simulink model "aquabot_main"  (R2023b)
settings: Solver=FixedStepAuto  StartTime=0.0  StopTime=Inf  RelTol=1e-3
model workspace (MAT data in the model file):
  SL_Bus_ROSEnable64bitIntegers = 1
  SL_ROS_VariableLengthArrays_MaxSizes.CommonInfo.ArrayTruncateAction = 'EmitWarning'
  SL_ROS_VariableLengthArrays_MaxSizes.MsgTypeMap = containers.Map
  SL_ROS_VariableLengthArrays_MaxSizes.MsgTypeMap.serialization.keys = {'nav_msgs/OccupancyGrid', 'sensor_msgs/Image', 'sensor_msgs/LaserScan', 'sensor_msgs/PointCloud2'}
  SL_ROS_VariableLengthArrays_MaxSizes.MsgTypeMap.serialization.values{1}.PropertyName = 'data'
  SL_ROS_VariableLengthArrays_MaxSizes.MsgTypeMap.serialization.values{1}.DataType = 'int8'
  SL_ROS_VariableLengthArrays_MaxSizes.MsgTypeMap.serialization.values{1}.MaxLength = 422500
  SL_ROS_VariableLengthArrays_MaxSizes.MsgTypeMap.serialization.values{2}(1).PropertyName = 'data'
  SL_ROS_VariableLengthArrays_MaxSizes.MsgTypeMap.serialization.values{2}(1).DataType = 'uint8'
  SL_ROS_VariableLengthArrays_MaxSizes.MsgTypeMap.serialization.values{2}(1).MaxLength = 1244160
  SL_ROS_VariableLengthArrays_MaxSizes.MsgTypeMap.serialization.values{2}(2).PropertyName = 'encoding'
  SL_ROS_VariableLengthArrays_MaxSizes.MsgTypeMap.serialization.values{2}(2).DataType = 'uint8'
  SL_ROS_VariableLengthArrays_MaxSizes.MsgTypeMap.serialization.values{2}(2).MaxLength = 1244160
  SL_ROS_VariableLengthArrays_MaxSizes.MsgTypeMap.serialization.values{3}(1).PropertyName = 'intensities'
  SL_ROS_VariableLengthArrays_MaxSizes.MsgTypeMap.serialization.values{3}(1).DataType = 'single'
  SL_ROS_VariableLengthArrays_MaxSizes.MsgTypeMap.serialization.values{3}(1).MaxLength = 1875
  SL_ROS_VariableLengthArrays_MaxSizes.MsgTypeMap.serialization.values{3}(2).PropertyName = 'ranges'
  SL_ROS_VariableLengthArrays_MaxSizes.MsgTypeMap.serialization.values{3}(2).DataType = 'single'
  SL_ROS_VariableLengthArrays_MaxSizes.MsgTypeMap.serialization.values{3}(2).MaxLength = 1875
  SL_ROS_VariableLengthArrays_MaxSizes.MsgTypeMap.serialization.values{4}(1).PropertyName = 'data'
  SL_ROS_VariableLengthArrays_MaxSizes.MsgTypeMap.serialization.values{4}(1).DataType = 'uint8'
  SL_ROS_VariableLengthArrays_MaxSizes.MsgTypeMap.serialization.values{4}(1).MaxLength = 960000
  SL_ROS_VariableLengthArrays_MaxSizes.MsgTypeMap.serialization.values{4}(2).PropertyName = 'fields'
  SL_ROS_VariableLengthArrays_MaxSizes.MsgTypeMap.serialization.values{4}(2).DataType = 'sensor_msgs/PointField'
  SL_ROS_VariableLengthArrays_MaxSizes.MsgTypeMap.serialization.values{4}(2).MaxLength = 16
  SL_ROS_VariableLengthArrays_MaxSizes.MsgTypeMap.serialization.uniformity = 0
  SL_ROS_VariableLengthArrays_MaxSizes.MsgTypeMap.serialization.keyType = 'char'
  SL_ROS_VariableLengthArrays_MaxSizes.MsgTypeMap.serialization.valueType = 'any'
undefined symbols (not defined in the file or in its folder): pose
libraries: ros2lib x16, simulink x1
settings Model: Creator=nicolas  LastModifiedBy=nicolas
settings OptimizationCC: EnhancedBackFolding=on  PassReuseOutputArgsAs=Individual arguments  ZeroExternalMemoryAtStartup=off  ZeroInternalMemoryAtStartup=off  MaxStackSize=64  OptimizeBlockOrder=speed  DifferentSizesBufferReuse=on  OptimizationCustomize=off  EfficientTunableParamExpr=on
settings DebuggingCC: ParameterTunabilityLossMsg=error
settings HardwareCC: ProdBitPerLong=64  ProdLongLongMode=on  ProdHWDeviceType=Intel->x86-64 (Linux 64)  UseEmbeddedCoderFeatures=off
settings SFSimCC: SimHardwareAcceleration=native  SimTargetLang=C++  SimGPUStackLimitPerThread=2048
settings RTWCC: Description=Embedded Coder  SystemTargetFile=ert.tlc  HardwareBoard=Robot Operating System 2 (ROS 2)  TLCOptions="-aInlineSetEventsForThisBaseRateFcn=TLC_FALSE -aSuppressMultiTaskScheduler=TLC_FALSE  -aRateBasedStepFcn=0"  TemplateMakefile=ert_default_tmf  Toolchain=Colcon Tools  BuildConfiguration=Faster Runs  TargetLang=C++
settings CodeAppCC: ForceParamTrailComments=on  IgnoreCustomStorageClasses=off  OperatorAnnotations=on  SimulinkDataObjDesc=on  SFDataObjDesc=on  InsertBlockDesc=on
settings ERTTargetCC: CodeInterfacePackaging=C++ class  SupportNonInlinedSFcns=on  RootIOFormat=Structure reference

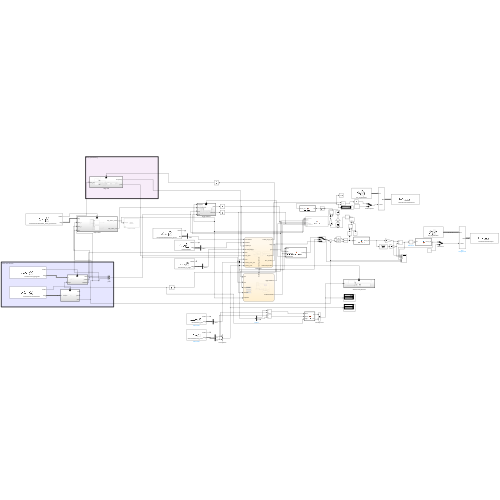
[thumbnail: Simulink's stored preview of the top-level diagram]
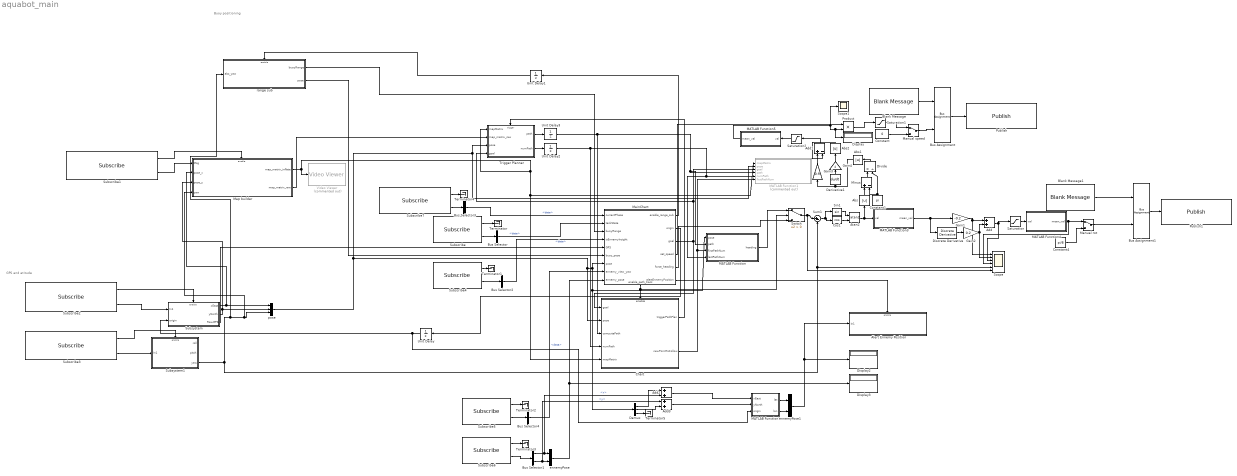
== system aquabot_main ==
  note: Buoy positioning
  note: GPS and atitude
  Abs : Abs  SaturateOnIntegerOverflow=off
  Abs1 : Abs  SaturateOnIntegerOverflow=off
  Abs2 : Abs  SaturateOnIntegerOverflow=off
  Add : Sum
  Add1 : Sum  Inputs=+-
  Add2 : Sum
  Add3 : Sum
  Alert Ennemy Position : Subsystem
  Atan2 : Trigonometry  Operator=atan2
  Blank Message : ros2lib/Blank Message  messageClass=Message  entityType=std_msgs/Float64  messageType=std_msgs/Float64  SampleTime=inf
  Blank Message1 : ros2lib/Blank Message  messageClass=Message  entityType=std_msgs/Float64  messageType=std_msgs/Float64  SampleTime=inf
  Bus Assignment : BusAssignment  AssignedSignals=data
  Bus Assignment1 : BusAssignment  AssignedSignals=data
  Bus Selector{,2..4} (4 alike) : BusSelector  OutputSignals=data
  Bus Selector1 : BusSelector  OutputSignals=pose.position.x,pose.position.y
  Chart : Stateflow chart  TreatAsAtomicUnit=on
      settings: PortSchema="{\"entries\":[{\"content\":{\"sides\":[{\"content\":{\"connectorIds\":[\"In2\",\"In3\",\"In4\",\"In5\",\"In6\"]},\"type\":\"ConnectorPlacement.EquallySpacedRectSide\",\"uuid\":\"f9d23542-f88c-4b93-885e-55d9e7a867a5\"},{\"content\":{\"connectorIds\":[\"Out1\",\"Out2\"],\"side\":\"RIGHT\"},\"type\":\"ConnectorPlacement.EquallySpacedRectSide\",\"uuid\":\"ec7f353a-44e5-4b1c-b599-993baee30662\"},{\"content\":{\"connectorIds\":[\"In1\"],\"side\":\"TOP\"},\"type\":\"ConnectorPlacement.EquallySpacedRectSide\",\"uuid\":\"e2b72665-f6a6-46cc-93cf-7087a3433fd3\"}]},\"type\":\"ConnectorPlacement.EquallySpacedConnector\",\"uuid\":\"eb72d472-900e-4b4b-88a5-7b3bc966b645\"}],\"packageUris\":[\"http://schema.mathworks.com/mf0/Connector/R2020b\"],\"version\":\"1.0\"}"
  Constant : Constant  Value=0
  Constant1 : Constant  Value=pi
  Constant4 : Constant  Value=pi/8
  Cos1 : Trigonometry  Operator=cos
  Demux : Demux  Outputs=3
  Derivative1 : Derivative
  Discrete Derivative : simulink/Discrete/Discrete Derivative  gainval=1.0  ICPrevScaledInput=0.0  OutMin=[]  OutMax=[]  OutDataType=fixdt(1, 16)  OutScaling=2^-10  DoSatur=off
  Display : Display
  Display2 : Display
  Display3 : Display
  Divide : Product  Inputs=*/  RndMeth=Zero  SaturateOnIntegerOverflow=on
  Gain1 : Gain  Gain=-0.2
  Gain2 : Gain  Gain=0.2
  Gain3 : Gain  Gain=0.9
  Gain4 : Gain  Gain=4
  MATLAB Function : MATLAB Function  TreatAsAtomicUnit=on
  MATLAB Function1 : MATLAB Function  Commented=on  TreatAsAtomicUnit=on
  MATLAB Function2 : MATLAB Function  TreatAsAtomicUnit=on
  MATLAB Function3 : MATLAB Function  TreatAsAtomicUnit=on
  MATLAB Function4 : MATLAB Function  TreatAsAtomicUnit=on
  MATLAB Function5 : MATLAB Function  TreatAsAtomicUnit=on
  MainChart : Stateflow chart  TreatAsAtomicUnit=on
      settings: PortSchema="{\"entries\":[{\"content\":{\"sides\":[{\"content\":{\"connectorIds\":[\"In9\",\"In1\",\"In2\",\"In3\",\"In4\",\"In5\",\"In6\",\"In7\",\"In8\"]},\"type\":\"ConnectorPlacement.EquallySpacedRectSide\",\"uuid\":\"baf46242-21ef-496b-8046-9b9a77bd2dcf\"},{\"content\":{\"connectorIds\":[\"Out1\",\"Out2\",\"Out3\",\"Out4\",\"Out6\",\"Out7\"],\"side\":\"RIGHT\"},\"type\":\"ConnectorPlacement.EquallySpacedRectSide\",\"uuid\":\"0a7db7ae-9b8c-430e-84d2-7611729502e6\"},{\"content\":{\"side\":\"TOP\"},\"type\":\"ConnectorPlacement.EquallySpacedRectSide\",\"uuid\":\"959f44e0-4ee3-46d3-b72a-0b37b61c16dd\"},{\"content\":{\"connectorIds\":[\"Out5\"],\"side\":\"BOTTOM\"},\"type\":\"ConnectorPlacement.EquallySpacedRectSide\",\"uuid\":\"d94f5cc5-2498-45e0-a229-1de127971452\"}]},\"type\":\"ConnectorPlacement.EquallySpacedConnector\",\"uuid\":\"f5cd4cf7-e63f-491e-bc4b-a2135ba07ed7\"}],\"packageUris\":[\"http://schema.mathworks.com/mf0/Connector/R2020b\"],\"version\":\"1.0\"}"
  Manual rot : ManualSwitch
  Manual speed : ManualSwitch
  Map builder : Subsystem
  Minus : Sum  Inputs=+-
  Product : Product
  Publish : ros2lib/Publish  topicSource=Select from ROS network  topic=/wamv/thrusters/main/thrust  messageType=std_msgs/Float64  QOSHistory=Keep last  QOSDepth=1  QOSReliability=Reliable  QOSDurability=Volatile
  Publish1 : ros2lib/Publish  topicSource=Select from ROS network  topic=/wamv/thrusters/main/pos  messageType=std_msgs/Float64  QOSHistory=Keep last  QOSDepth=1  QOSReliability=Reliable  QOSDurability=Volatile
  Saturation : Saturate  UpperLimit=pi/4  LowerLimit=-pi/4
  Saturation1 : Saturate  UpperLimit=12000  LowerLimit=-12000
  Saturation2 : Saturate  UpperLimit=1  LowerLimit=0.1
  Scope : Scope  NumInputPorts=6
  Scope1 : Scope
  Sin1 : Trigonometry
  Subscribe : ros2lib/Subscribe  topicSource=Select from ROS network  topic=/siera/task/state  messageType=std_msgs/Int64  sampleTime=-1  QOSHistory=Keep last  QOSDepth=1  QOSReliability=Reliable  QOSDurability=Volatile
  Subscribe1 : ros2lib/Subscribe  topicSource=Select from ROS network  topic=/wamv/sensors/lidars/lidar_wamv_sensor/scan  messageType=sensor_msgs/LaserScan  sampleTime=-1  QOSHistory=Keep last  QOSDepth=1  QOSReliability=Reliable  QOSDurability=Volatile
  Subscribe2 : ros2lib/Subscribe  topicSource=Select from ROS network  topic=/wamv/sensors/gps/gps/fix  messageType=sensor_msgs/NavSatFix  sampleTime=-1  QOSHistory=Keep last  QOSDepth=1  QOSReliability=Reliable  QOSDurability=Volatile
  Subscribe3 : ros2lib/Subscribe  topicSource=Select from ROS network  topic=/wamv/sensors/imu/imu/data  messageType=sensor_msgs/Imu  sampleTime=-1  QOSHistory=Keep last  QOSDepth=1  QOSReliability=Reliable  QOSDurability=Volatile
  Subscribe4 : ros2lib/Subscribe  topicSource=Select from ROS network  topic=/siera/view/is_in_sight  messageType=std_msgs/Bool  sampleTime=-1  QOSHistory=Keep last  QOSDepth=1  QOSReliability=Reliable  QOSDurability=Volatile
  Subscribe5 : ros2lib/Subscribe  topicSource=Select from ROS network  topic=/siera/view/rel_yaw  messageType=std_msgs/Float64  sampleTime=-1  QOSHistory=Keep last  QOSDepth=1  QOSReliability=Reliable  QOSDurability=Volatile
  Subscribe6 : ros2lib/Subscribe  topicSource=Select from ROS network  topic=/siera/view/ennemy_pose  messageType=geometry_msgs/PoseStamped  sampleTime=-1  QOSHistory=Keep last  QOSDepth=1  QOSReliability=Reliable  QOSDurability=Volatile
  Subscribe7 : ros2lib/Subscribe  topicSource=Select from ROS network  topic=/vrx/patrolandfollow/current_phase  messageType=std_msgs/UInt32  sampleTime=-1  QOSHistory=Keep last  QOSDepth=1  QOSReliability=Reliable  QOSDurability=Volatile
  Subsystem : Subsystem
  Subsystem1 : Subsystem
  Sum1 : Sum  Inputs=|+-
  Switch : Switch  Criteria=u2 > Threshold  SaturateOnIntegerOverflow=off  InputSameDT=off
  Terminator{,1..5} (6 alike) : Terminator
  Trigger Planner : Subsystem
  Unit Delay : UnitDelay  InitialCondition=[0 0]  SampleTime=-1  HasFrameUpgradeWarning=on
  Unit Delay1 : UnitDelay  SampleTime=-1  HasFrameUpgradeWarning=on
  Unit Delay2 : UnitDelay  SampleTime=-1  HasFrameUpgradeWarning=on
  Unit Delay3 : UnitDelay  InitialCondition=zeros(100,3)  SampleTime=-1  HasFrameUpgradeWarning=on
  Video Viewer : VideoViewer  Commented=on  FigPos=[317 969 1054 739]
  ennemyPose : Concatenate
  ennemyPose1 : Concatenate
  pose : Concatenate  NumInputs=3
  range sub : Subsystem
  wires:
  Subscribe1/2 -> Map builder/1(Msg)
  Subscribe1/1 -> Map builder/Enable
  Subscribe3/2 -> Subsystem1/1(In1)
  Subscribe3/1 -> Subsystem1/Enable
  Map builder/1(map_matrix_inflate) -> Video Viewer/1, Trigger Planner/1(mapMatrix), Chart/6(mapMatrix), MATLAB Function1/1(mapMatrix)
  Subscribe4/2 -> Bus Selector2/1
  Bus Selector/1 -> MainChart/1(taskState)  "<data>"
  MainChart/1(enable_range_sub) -> Unit Delay1/1
  Blank Message/1 -> Bus Assignment/1
  Bus Assignment/1 -> Publish/1
  Subscribe2/2 -> Subsystem/1(In1)
  MainChart/2(origin) -> Unit Delay/1
  Subsystem/3(RawGPS) -> MainChart/4(GPS)
  Subscribe2/1 -> Subsystem/Enable
  Unit Delay/1 -> MATLAB Function2/3(origin), Subsystem/2(origin)
  Subsystem/1(xEast) -> Map builder/2(pose_x), pose/1
  Subsystem/2(yNorth) -> pose/2, Map builder/3(pose_y)
  pose/1 -> MATLAB Function1/2(pose), Trigger Planner/3(pose), Chart/3(pose), Demux/1, MATLAB Function/1(pose), MainChart/6(pose)
  Unit Delay1/1 -> range sub/Enable
  range sub/2(pose) -> MainChart/5(buoy_pose)
  Trigger Planner/2(numPath) -> Unit Delay2/1
  Chart/1(triggerPathPlan) -> Trigger Planner/Trigger
  Trigger Planner/1(path) -> Unit Delay3/1
  Unit Delay2/1 -> Chart/5(numPath), MATLAB Function1/5(numPath), MATLAB Function/4(lastPathNum)
  Unit Delay3/1 -> Chart/4(computePath), MATLAB Function/2(path), MATLAB Function1/4(path)
  Chart/2(newPointToFollow) -> MATLAB Function/3(firstPathNum), MATLAB Function1/6(firstPathNum)
  Blank Message1/1 -> Bus Assignment1/1
  Bus Assignment1/1 -> Publish1/1
  MATLAB Function/1(heading) -> Switch/1
  MATLAB Function3/1(mean_val) -> Gain1/1, Discrete Derivative/1
  Cos1/1 -> Atan2/2
  Sin1/1 -> Atan2/1
  Atan2/1 -> MATLAB Function3/1(val), Abs/1
  Sum1/1 -> Sin1/1, Cos1/1
  Gain2/1 -> Scope/2, Add/2
  Gain1/1 -> Add/1, Scope/1
  Saturation/1 -> MATLAB Function4/1(val)
  Add/1 -> Saturation/1, Scope/3
  MainChart/4(set_speed) -> Product/1
  Manual speed/1 -> Bus Assignment/2
  Constant/1 -> Manual speed/2
  Constant4/1 -> Manual rot/2
  Manual rot/1 -> Bus Assignment1/2
  Subsystem1/3(yaw) -> pose/3, Map builder/4(yaw), range sub/1(abs_yaw), Sum1/2, Scope/5
  range sub/1(buoyRange) -> MainChart/2(buoyRange)
  MainChart/3(goal) -> Chart/2(goal), MATLAB Function1/3(goal), Trigger Planner/4(goal)
  MainChart/5(enable_path_track) -> Switch/2, Chart/1(enable)
  Abs/1 -> Minus/1
  Constant1/1 -> Minus/2, Divide/2
  Minus/1 -> Divide/1
  Divide/1 -> Abs1/1
  Saturation1/1 -> Manual speed/1
  Product/1 -> Saturation1/1
  MATLAB Function5/1(mean_val) -> Display/1, Product/2, Scope1/1
  Derivative1/1 -> Gain4/1
  Add1/1 -> Saturation2/1
  Gain3/1 -> Add1/1
  Abs1/1 -> Gain3/1, Derivative1/1
  Gain4/1 -> Abs2/1
  Abs2/1 -> Add1/2
  Subscribe/2 -> Bus Selector/1
  Subscribe/1 -> Terminator/1
  Switch/1 -> Scope/6, Sum1/1
  MainChart/6(force_heading) -> Switch/3
  Subscribe4/1 -> Terminator1/1
  Subscribe5/1 -> Terminator2/1
  Subscribe6/2 -> Bus Selector1/1
  Subscribe6/1 -> Terminator3/1
  Bus Selector1/2 -> Add3/1, ennemyPose/2  "<y>"
  Bus Selector1/1 -> Add2/2, ennemyPose/1  "<x>"
  Subscribe5/2 -> Bus Selector4/1
  ennemyPose/1 -> Display3/1, MainChart/8(ennemy_pose)
  Subscribe7/1 -> Terminator4/1
  Subscribe7/2 -> Bus Selector3/1
  MainChart/7(alertEnnemyPosition) -> Alert Ennemy Position/Enable
  Bus Selector2/1 -> MainChart/3(isEnnemyInsight)  "<data>"
  Bus Selector3/1 -> MainChart/9(currentPhase)  "<data>"
  Bus Selector4/1 -> MainChart/7(ennemy_view_yaw)  "<data>"
  MATLAB Function2/1(lat) -> ennemyPose1/1
  MATLAB Function2/2(lon) -> ennemyPose1/2
  ennemyPose1/1 -> Alert Ennemy Position/1(In1), Display2/1
  MATLAB Function4/1(mean_val) -> Scope/4, Manual rot/1
  Discrete Derivative/1 -> Gain2/1
  Saturation2/1 -> MATLAB Function5/1(val)
  Add2/1 -> MATLAB Function2/1(xEast)
  Add3/1 -> MATLAB Function2/2(yNorth)
  Demux/1 -> Add2/1
  Demux/2 -> Add3/2
  Demux/3 -> Terminator5/1
  Map builder/2(map_matrix_raw) -> Trigger Planner/2(map_matrix_raw)

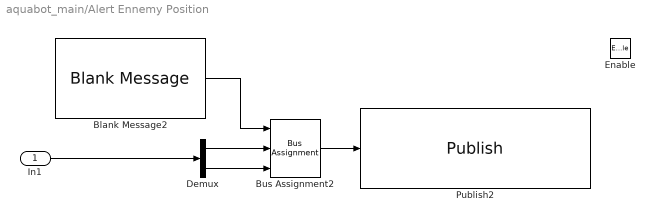
== system aquabot_main/Alert Ennemy Position ==
  In1 : Inport
  Enable : EnablePort
  Blank Message2 : ros2lib/Blank Message  messageClass=Message  entityType=geometry_msgs/PoseStamped  messageType=geometry_msgs/PoseStamped  SampleTime=inf
  Bus Assignment2 : BusAssignment  AssignedSignals=pose.position.x,pose.position.y
  Demux : Demux  Outputs=2
  Publish2 : ros2lib/Publish  topicSource=Select from ROS network  topic=/vrx/patrolandfollow/alert_position  messageType=geometry_msgs/PoseStamped  QOSHistory=Keep last  QOSDepth=1  QOSReliability=Reliable  QOSDurability=Volatile
  wires:
  In1/1 -> Demux/1
  Demux/1 -> Bus Assignment2/2
  Bus Assignment2/1 -> Publish2/1
  Blank Message2/1 -> Bus Assignment2/1
  Demux/2 -> Bus Assignment2/3

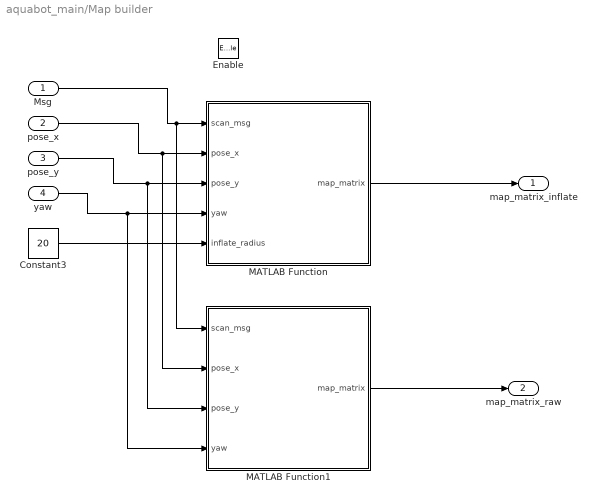
== system aquabot_main/Map builder ==
  Msg : Inport
  pose_x : Inport  Port=2
  pose_y : Inport  Port=3
  yaw : Inport  Port=4
  Enable : EnablePort
  Constant3 : Constant  Value=20
  MATLAB Function : MATLAB Function  TreatAsAtomicUnit=on
  MATLAB Function1 : MATLAB Function  TreatAsAtomicUnit=on
  map_matrix_inflate : Outport
  map_matrix_raw : Outport  Port=2
  wires:
  Msg/1 -> MATLAB Function1/1(scan_msg), MATLAB Function/1(scan_msg)
  MATLAB Function/1(map_matrix) -> map_matrix_inflate/1
  pose_x/1 -> MATLAB Function1/2(pose_x), MATLAB Function/2(pose_x)
  pose_y/1 -> MATLAB Function1/3(pose_y), MATLAB Function/3(pose_y)
  yaw/1 -> MATLAB Function1/4(yaw), MATLAB Function/4(yaw)
  Constant3/1 -> MATLAB Function/5(inflate_radius)
  MATLAB Function1/1(map_matrix) -> map_matrix_raw/1

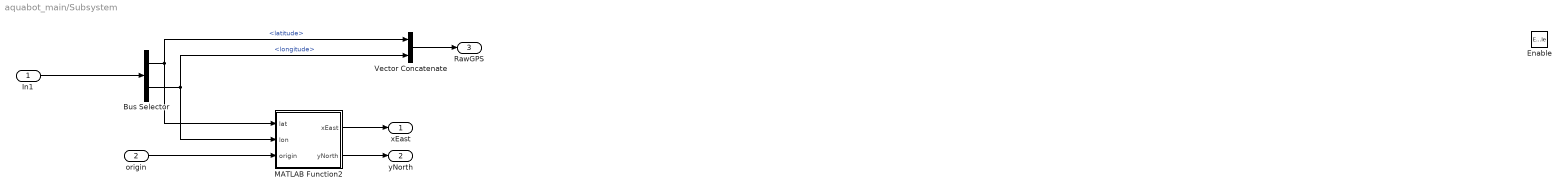
== system aquabot_main/Subsystem ==
  In1 : Inport
  origin : Inport  Port=2
  Enable : EnablePort
  Bus Selector : BusSelector  OutputSignals=latitude,longitude
  MATLAB Function2 : MATLAB Function  TreatAsAtomicUnit=on
  Vector Concatenate : Concatenate
  xEast : Outport
  yNorth : Outport  Port=2
  RawGPS : Outport  Port=3
  wires:
  In1/1 -> Bus Selector/1
  Bus Selector/1 -> MATLAB Function2/1(lat), Vector Concatenate/1  "<latitude>"
  Vector Concatenate/1 -> RawGPS/1
  Bus Selector/2 -> MATLAB Function2/2(lon), Vector Concatenate/2  "<longitude>"
  origin/1 -> MATLAB Function2/3(origin)
  MATLAB Function2/1(xEast) -> xEast/1
  MATLAB Function2/2(yNorth) -> yNorth/1

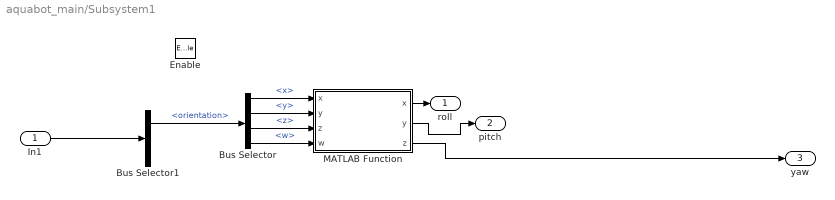
== system aquabot_main/Subsystem1 ==
  In1 : Inport
  Enable : EnablePort
  Bus Selector : BusSelector  OutputSignals=x,y,z,w
  Bus Selector1 : BusSelector  OutputSignals=orientation,angular_velocity
  MATLAB Function : MATLAB Function  TreatAsAtomicUnit=on
  roll : Outport
  pitch : Outport  Port=2
  yaw : Outport  Port=3
  wires:
  Bus Selector1/1 -> Bus Selector/1  "<orientation>"
  Bus Selector/2 -> MATLAB Function/2("y ")  "<y>"
  Bus Selector/4 -> MATLAB Function/4(w)  "<w>"
  Bus Selector/3 -> MATLAB Function/3("z ")  "<z>"
  MATLAB Function/2(y) -> pitch/1
  Bus Selector/1 -> MATLAB Function/1("x ")  "<x>"
  In1/1 -> Bus Selector1/1
  MATLAB Function/3(z) -> yaw/1
  MATLAB Function/1(x) -> roll/1

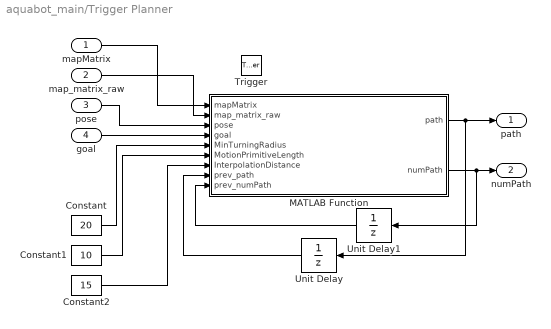
== system aquabot_main/Trigger Planner ==
  mapMatrix : Inport
  map_matrix_raw : Inport  Port=2
  pose : Inport  Port=3
  goal : Inport  Port=4
  Trigger : TriggerPort  VariantControl=(inherit)  PortDimensions=1
  Constant : Constant  Value=20
  Constant1 : Constant  Value=10
  Constant2 : Constant  Value=15
  MATLAB Function : MATLAB Function  TreatAsAtomicUnit=on
  Unit Delay : UnitDelay  InitialCondition=zeros(100,3)  SampleTime=-1  HasFrameUpgradeWarning=on
  Unit Delay1 : UnitDelay  InitialCondition=1  SampleTime=-1  HasFrameUpgradeWarning=on
  path : Outport
  numPath : Outport  Port=2
  wires:
  goal/1 -> MATLAB Function/4(goal)
  pose/1 -> MATLAB Function/3(pose)
  MATLAB Function/2(numPath) -> Unit Delay1/1, numPath/1
  mapMatrix/1 -> MATLAB Function/1(mapMatrix)
  MATLAB Function/1(path) -> Unit Delay/1, path/1
  Constant2/1 -> MATLAB Function/7(InterpolationDistance)
  Constant1/1 -> MATLAB Function/6(MotionPrimitiveLength)
  Constant/1 -> MATLAB Function/5(MinTurningRadius)
  Unit Delay/1 -> MATLAB Function/8(prev_path)
  Unit Delay1/1 -> MATLAB Function/9(prev_numPath)
  map_matrix_raw/1 -> MATLAB Function/2(map_matrix_raw)

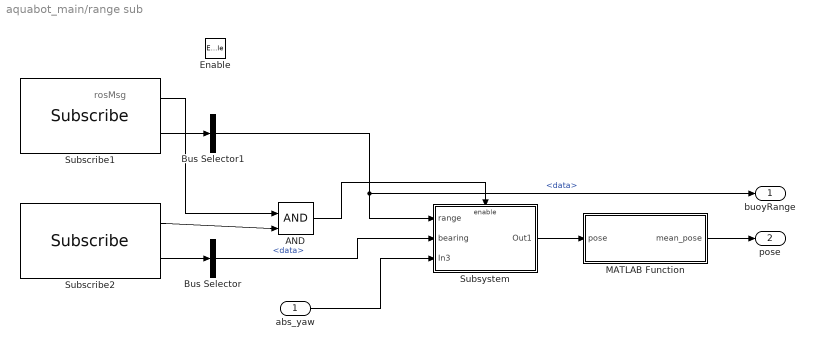
== system aquabot_main/range sub ==
  note: rosMsg
  abs_yaw : Inport
  Enable : EnablePort
  AND : Logic  IconShape=distinctive  AllPortsSameDT=off  OutDataTypeStr=boolean
  Bus Selector : BusSelector  OutputSignals=data
  Bus Selector1 : BusSelector  OutputSignals=data
  MATLAB Function : MATLAB Function  TreatAsAtomicUnit=on
  Subscribe1 : ros2lib/Subscribe  topicSource=Select from ROS network  topic=/siera/pinger/range  messageType=std_msgs/Float64  sampleTime=-1  QOSHistory=Keep last  QOSDepth=1  QOSReliability=Reliable  QOSDurability=Volatile
  Subscribe2 : ros2lib/Subscribe  topicSource=Select from ROS network  topic=/siera/pinger/bearing  messageType=std_msgs/Float64  sampleTime=-1  QOSHistory=Keep last  QOSDepth=1  QOSReliability=Reliable  QOSDurability=Volatile
  Subsystem : Subsystem
  buoyRange : Outport
  pose : Outport  Port=2
  wires:
  Subscribe1/2 -> Bus Selector1/1
  Subscribe2/2 -> Bus Selector/1
  Subscribe2/1 -> AND/2
  Subscribe1/1 -> AND/1
  Bus Selector1/1 -> buoyRange/1, Subsystem/1(range)  "<data>"
  Bus Selector/1 -> Subsystem/2(bearing)  "<data>"
  abs_yaw/1 -> Subsystem/3(In3)
  Subsystem/1(Out1) -> MATLAB Function/1(pose)
  AND/1 -> Subsystem/Enable
  MATLAB Function/1(mean_pose) -> pose/1

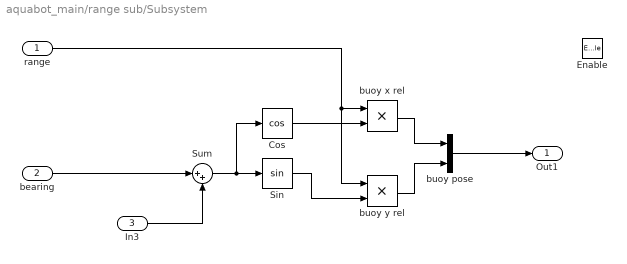
== system aquabot_main/range sub/Subsystem ==
  range : Inport
  bearing : Inport  Port=2
  In3 : Inport  Port=3
  Enable : EnablePort
  Cos : Trigonometry  Operator=cos
  Sin : Trigonometry
  Sum : Sum  Inputs=|++
  buoy pose : Concatenate
  buoy x rel : Product
  buoy y rel : Product
  Out1 : Outport
  wires:
  Cos/1 -> buoy x rel/2
  In3/1 -> Sum/2
  buoy pose/1 -> Out1/1
  Sin/1 -> buoy y rel/2
  buoy x rel/1 -> buoy pose/1
  buoy y rel/1 -> buoy pose/2
  range/1 -> buoy y rel/1, buoy x rel/1
  Sum/1 -> Cos/1, Sin/1
  bearing/1 -> Sum/1

== matlab function aquabot_main/Map builder/MATLAB Function ==
  data: scan_msg input; map_matrix output; pose_x input; pose_y input; yaw input; inflate_radius input
function map_matrix= fcn(scan_msg, pose_x, pose_y, yaw,inflate_radius)
    ranges = scan_msg.ranges;
    ranges(ranges==inf) = NaN;
    angles = transpose(linspace(scan_msg.angle_min, scan_msg.angle_max, length(ranges)));

    map = binaryOccupancyMap(700, 700,1);
    map.GridOriginInLocal = -[diff(map.XWorldLimits) diff(map.YWorldLimits)]/2;
    insertRay(map, [pose_x pose_y yaw], ranges, angles, 130);
    inflate(map,inflate_radius)
    map_matrix = map.occupancyMatrix();
end

== matlab function aquabot_main/Subsystem1/MATLAB Function ==
  data: x output; x input; y output; y input; z input; w input; z output
function [x, y, z]= quatToEuler(x, y, z, w)
    eulZYX = quat2eul([w, x, y, z], "ZYX");
    x = eulZYX(3);
    y = eulZYX(2);
    z = eulZYX(1);
end

== stateflow chart aquabot_main/MainChart ==
  state Init
    entry:
    goal = [0; 0];
    set_speed=0;
    enable_path_track = 0;
    force_heading = pose(3);
    listOfPoints = [[200;200],[200;-200],[0;200],[0;-200],[-200;200],[-200;-200]];
  state SeekBuoy
    entry:
    origin = [GPS(1); GPS(2)];
    force_heading = pose(3);
    enable_range_sub=1;
    set_speed=8000;
    enable_path_track = 1;
    during:
    new_goal = [buoy_pose(1) + pose(1); buoy_pose(2) + pose(2)];
    goal = (new_goal + goal) / 2;
  state FineBuoySeeking
    entry:
    set_speed=2000;
    force_heading = pose(3);
    enable_path_track = 0;
    during:
    force_heading = atan2(goal(2)-pose(2), goal(1)-pose(1));
  state BuoyFound
    entry:
    set_speed=2000;
    force_heading = pose(3);
    enable_path_track = 0;
    during:
    force_heading = atan2(-goal(2)-pose(2), -goal(1)-pose(1));
  state Patroll
    entry:
    set_speed=0;
    enable_range_sub=0;
    state Init
    state FollowGoal
      entry:
      set_speed=10000;
      goal = listOfPoints(:,indexOfNextGoal);
      enable_path_track = 1;
    state GoalAchieve
      entry:
      indexOfNextGoal = mod(indexOfNextGoal, size(listOfPoints,2))+1;
    (default) -> Patroll.Init
    Patroll.Init -> FollowGoal
    GoalAchieve -> FollowGoal
    FollowGoal -> GoalAchieve : [norm(goal - pose(1:2)) <= 10]
  state SeekEnnemy
    entry:
    set_speed=0;
    state SeekInSight
      entry:
      set_speed=5000;
      enable_path_track = 1;
      during:
      force_heading = pose(3) - ennemy_view_yaw;
      goal = pose(1:2) + [80 * cos(pose(3) - ennemy_view_yaw); 80*sin(pose(3)) - ennemy_view_yaw ];
    state SearchLastKnowZone
      set_speed=3000;
      enable_path_track = 1;
    state EnnemyOnLidar
      entry:
      enable_path_track = 1;
      alertEnnemyPosition=1;
      during:
      % force_heading = pose(3) - ennemy_view_yaw;
      goal = pose(1:2) + ennemy_pose;
      distance = norm(goal - pose(1:2));
      set_speed = max(min((distance-30)*30,3000),0);
    (default) -> SeekInSight
    SeekInSight -> SearchLastKnowZone [order 1] : [isEnnemyInsight==0]
    (junction 177) -> SeekInSight [order 1] : [isEnnemyInsight==1]
    SearchLastKnowZone -> SeekInSight [order 2] : [isEnnemyInsight==1]
    SeekInSight -> EnnemyOnLidar [order 2] : [all(ennemy_pose)~=0]
    SearchLastKnowZone -> EnnemyOnLidar [order 1] : [all(ennemy_pose)~=0]
    SearchLastKnowZone -> (junction 177) [order 3] : [norm(goal - pose(1:2)) <= 5]
    EnnemyOnLidar -> SearchLastKnowZone : [all(ennemy_pose)==0]{alertEnnemyPosition=0;}
  state TurnAroundToSeekNearEnnemy
    entry:
    start_yaw = pose(3);
    force_heading = start_yaw;
    during:
    force_heading = force_heading + 0.002;
  (default) -> Init
  Init -> SeekBuoy : [taskState==2 && all(GPS)~=0]
  SeekBuoy -> FineBuoySeeking : [buoyRange<=40||currentPhase>=2]
  FineBuoySeeking -> BuoyFound : [buoyRange<=20||currentPhase>=2]
  Patroll -> SeekEnnemy : [isEnnemyInsight==1]
  TurnAroundToSeekNearEnnemy -> Patroll [order 1] : [force_heading-start_yaw>=2*pi]
  BuoyFound -> TurnAroundToSeekNearEnnemy : [currentPhase>=2]{indexOfNextGoal = 1;}
  (junction 177) -> TurnAroundToSeekNearEnnemy [order 2] : after(50,sec)
  TurnAroundToSeekNearEnnemy -> SeekEnnemy [order 2] : [isEnnemyInsight==1]
  data: taskState input; buoyRange input; isEnnemyInsight input; enable_range_sub output; origin output; GPS input; buoy_pose input; pose input; goal output; new_goal local; set_speed output; enable_path_track output; force_heading output; listOfPoints local; indexOfNextGoal local; ennemy_view_yaw input; ennemy_pose input; alertEnnemyPosition output; currentPhase input; start_yaw local; distance local

== matlab function aquabot_main/MATLAB Function2 ==
  data: lat output; lon output; xEast input; yNorth input; origin input
function [lat,lon] = XY2GPS(xEast,yNorth, origin)
    earth_radius = 6371000.0;
    
    if all(origin == 0)
        lat = 0;
        lon = 0;
    else
        lat = rad2deg(asin(yNorth/earth_radius)) + origin(1);
        lon = rad2deg(asin(xEast/(earth_radius*cos(asin(yNorth/earth_radius))))) + origin(2);
    end
end

== matlab function aquabot_main/MATLAB Function3 ==
  data: val input; mean_val output
function mean_val = movMean(val)
    persistent vals;
    persistent lastValIndex;    
    mov_length = 10;
    
    if isempty(vals)
        vals = zeros(mov_length,1);
        lastValIndex = 1;
    end

    vals = circshift(vals, [-1 0]);
    vals(lastValIndex) = val;

    mean_val = mean(vals(1:lastValIndex,:));
    if lastValIndex < mov_length
        lastValIndex = lastValIndex + 1;
    end
end

== matlab function aquabot_main/Trigger Planner/MATLAB Function ==
  data: mapMatrix input; map_matrix_raw input; path output; numPath output; pose input; goal input; MinTurningRadius input; MotionPrimitiveLength input; InterpolationDistance input; prev_path input; prev_numPath input
function [path, numPath] = planner(mapMatrix, map_matrix_raw, pose, goal, MinTurningRadius, MotionPrimitiveLength, InterpolationDistance, prev_path, prev_numPath)
    persistent prev_goal;
    MaxPathNum = 100;

    if isempty(prev_goal)
        prev_goal = goal;
    end

    map = binaryOccupancyMap(mapMatrix, 1);
    map.GridOriginInLocal = -[diff(map.XWorldLimits) diff(map.YWorldLimits)]/2;
    
    ss = stateSpaceSE2;
    ss.StateBounds = [map.XWorldLimits;map.YWorldLimits;[-pi pi]];
    if isempty(ss)
        path = prev_path;
        numPath = prev_numPath;
        return;
    end
    sv = validatorOccupancyMap(ss,Map=map);

    planner = plannerHybridAStar(sv, MinTurningRadius=MinTurningRadius, MotionPrimitiveLength=MotionPrimitiveLength, InterpolationDistance=InterpolationDistance);
    startPose = pose'; % [meters, meters, radians]
    goal(1) = min(max(goal(1),-320),320);
    goal(2) = min(max(goal(2),-320),320);
    goalOrientation = atan2(goal(2) - pose(2), goal(1) - pose(1));
    goalPose = [goal(1) goal(2) goalOrientation];
    
    if ~isStateValid(sv,startPose)
        map = binaryOccupancyMap(map_matrix_raw, 1);
        map.GridOriginInLocal = -[diff(map.XWorldLimits) diff(map.YWorldLimits)]/2;
        sv = validatorOccupancyMap(ss,Map=map);
        planner = plannerHybridAStar(sv, MinTurningRadius=MinTurningRadius, MotionPrimitiveLength=MotionPrimitiveLength, InterpolationDistance=InterpolationDistance);
    end

    if ~isStateValid(sv,goalPose)
        [~, lastValid] = isMotionValid(sv,startPose,goalPose);
        goalOrientation = atan2(lastValid(2) - pose(2), lastValid(1) - pose(1));            
        goalPose = [lastValid(1) lastValid(2) goalOrientation];
    end

    if norm(startPose - goalPose) <= 10
        path = zeros(MaxPathNum,3);
        path(1,:) = startPose;
        goalOrientation = atan2(goal(2) - pose(2), goal(1) - pose(1));
        goalPose = [goal(1) goal(2) goalOrientation];
        path(2,:) = goalPose;
        numPath=2;
    else
        refpath = plan(planner,startPose,goalPose);
        path = zeros(MaxPathNum,3);
        path(1:refpath.NumStates,:) = refpath.States;
        numPath=refpath.NumStates;
    end
end

== matlab function aquabot_main/MATLAB Function1 ==
  data: mapMatrix input; pose input; goal input; path input; numPath input; firstPathNum input
function viewDebug(mapMatrix, pose, goal, path, numPath, firstPathNum)
    [r,c] = ind2sub(size(mapMatrix), find(mapMatrix));
    r = 325 - r;
    c = c - 325;
    
    hold off
    scatter(c,r,'filled','square','MarkerFaceColor','k')
    hold on
    plot(pose(1), pose(2), "-o", "MarkerEdgeColor", "g")
    plot(goal(1), goal(2), "-o", "MarkerEdgeColor", "r")
    range = 25;
    quiver(pose(1), pose(2), range*cos(pose(3)), range*sin(pose(3)))

    if numPath > 0
        scatter(path(firstPathNum+1:numPath-1,1),path(firstPathNum+1:numPath-1,2),'o','MarkerFaceColor','b')
        scatter(path(firstPathNum,1),path(firstPathNum,2),'o','MarkerFaceColor','g')
        scatter(path(numPath,1),path(numPath,2),'o','MarkerFaceColor','r')
        range = 5;
        quiver(path(firstPathNum:numPath,1), path(firstPathNum:numPath,2), range*cos(path(firstPathNum:numPath,3)), range*sin(path(firstPathNum:numPath,3)))
    end

    xlim([-325 325])
    ylim([-325 325])
end

== matlab function aquabot_main/Subsystem/MATLAB Function2 ==
  data: xEast output; yNorth output; lat input; lon input; origin input
function [xEast,yNorth] = GPS2XY(lat,lon, origin)
    earth_radius = 6371000.0;
    
    if all(origin == 0)
        xEast = 0;
        yNorth = 0;
    else
        xEast = earth_radius * cos(deg2rad(lat - origin(1))) * sin(deg2rad(lon - origin(2)));
        yNorth = earth_radius * sin(deg2rad(lat - origin(1)));
    end
end

== matlab function aquabot_main/MATLAB Function ==
  data: pose input; path input; heading output; firstPathNum input; lastPathNum input
function heading = convertPathPlanToHeading(pose, path, firstPathNum, lastPathNum)
    persistent prev_heading;
    if isempty(prev_heading)
        prev_heading = pose(3);
    end

    if lastPathNum == 0
        heading = pose(3);
    else
        if firstPathNum+1 > lastPathNum
            heading = pose(3);
        else
            point = path(firstPathNum+1,:);
            heading = atan2(point(2)-pose(2), point(1)-pose(1));
            heading_jump = abs(heading - prev_heading);
            if heading_jump >= 0.05
                if heading_jump <= 2
                    heading = (heading + prev_heading) / 2;
                else
                    heading = pose(3);
                end
            end
        end
    end
    prev_heading = heading;
end

== matlab function aquabot_main/MATLAB Function4 ==
  data: val input; mean_val output
function mean_val = movMean(val)
    persistent vals;
    persistent lastValIndex;    
    mov_length = 5;
    
    if isempty(vals)
        vals = zeros(mov_length,1);
        lastValIndex = 1;
    end

    vals = circshift(vals, [-1 0]);
    vals(lastValIndex) = val;

    mean_val = mean(vals(1:lastValIndex,:));
    if lastValIndex < mov_length
        lastValIndex = lastValIndex + 1;
    end
end

== matlab function aquabot_main/range sub/MATLAB Function ==
  data: pose input; mean_pose output
function mean_pose = poseMovMean(pose)
    persistent poses;
    persistent lastPosesIndex;    
    mov_length = 30;
    
    if isempty(poses)
        poses = zeros(mov_length, 2);
        lastPosesIndex = 1;
    end

    poses = circshift(poses, [-1 0]);
    poses(lastPosesIndex, :) = pose;

    mean_pose = mean(poses(1:lastPosesIndex,:), 1);
    if lastPosesIndex < mov_length
        lastPosesIndex = lastPosesIndex + 1;
    end
end

== stateflow chart aquabot_main/Chart ==
  state StandBy
    triggerPathPlan = 0;
  state TriggerPathPlan
    entry:
    triggerPathPlan = 1;
    newPointToFollow = 1;
  state UntriggerPathPlan
    entry:
    triggerPathPlan = 0;
  state CheckIfPathIsStillValid
    entry:
    pathIsValid = checkIfPathIsValid();
  state FollowPathPlan
  state DeleteNearNode
    entry:
    newPointToFollow = newPointToFollow+1;
  (default) -> StandBy
  (junction 2) -> StandBy
  (junction 58) -> (junction 2)
  StandBy -> TriggerPathPlan : [enable==1]
  TriggerPathPlan -> UntriggerPathPlan : after(1,sec)
  FollowPathPlan -> TriggerPathPlan [order 1] : [DistanceFromPathGoalToRealGoal() >= 20||DistanceFromPoseToFirstPathPoint() >= 20]
  UntriggerPathPlan -> FollowPathPlan
  CheckIfPathIsStillValid -> TriggerPathPlan [order 2] : [pathIsValid==0]
  FollowPathPlan -> (junction 58) [order 4] : [enable==0]
  CheckIfPathIsStillValid -> FollowPathPlan [order 1] : [pathIsValid==1]
  (junction 6) -> (junction 58)
  FollowPathPlan -> CheckIfPathIsStillValid [order 3] : after(1,sec)
  FollowPathPlan -> DeleteNearNode [order 2] : [DistanceFromPoseToFirstPathPoint() <= 5]
  DeleteNearNode -> FollowPathPlan [order 1] : [newPointToFollow<numPath]
  DeleteNearNode -> (junction 6) [order 2] : [newPointToFollow>=numPath]
  data: dist function_output; dist function_output; b function_output; enable input; triggerPathPlan output; newPointToFollow output; goal input; pose input; computePath input; numPath input; mapMatrix input; pathIsValid local
  function dist = DistanceFromPoseToFirstPathPoint:
    | function dist = DistanceFromPoseToFirstPathPoint()
    |     if numPath <= newPointToFollow+1
    |         dist = 0;
    |     else
    |         pathGoal2D = computePath(newPointToFollow+1, 1:2);
    |         dist = norm(pathGoal2D' - pose(1:2));
    |     end
    | end
  function dist = DistanceFromPathGoalToRealGoal:
    | function dist = DistanceFromPathGoalToRealGoal()
    |     if numPath > 0
    |         pathGoal2D = computePath(numPath, 1:2);
    |         dist = norm(pathGoal2D' - goal);
    |     else
    |         dist = Inf;
    |     end
    | end
  function b = checkIfPathIsValid:
    | function b = checkIfPathIsValid()
    |     map = binaryOccupancyMap(mapMatrix, 1);
    |     map.GridOriginInLocal = -[diff(map.XWorldLimits) diff(map.YWorldLimits)]/2;
    |     
    |     ss = stateSpaceSE2;
    |     ss.StateBounds = [map.XWorldLimits;map.YWorldLimits;[-pi pi]];
    |     sv = validatorOccupancyMap(ss,Map=map);
    | 
    |     b = 1;
    |     for i = newPointToFollow:numPath-1
    |         [isPathValid, lastValid] = isMotionValid(sv,computePath(i,:),computePath(i+1,:));
    |         if ~isPathValid
    |             b = 0;
    |             return
    |         end
    |     end
    | end

== matlab function aquabot_main/MATLAB Function5 ==
  data: val input; mean_val output
function mean_val = movMean(val)
    persistent vals;
    persistent lastValIndex;    
    mov_length = 10;
    
    if isempty(vals)
        vals = zeros(mov_length,1);
        lastValIndex = 1;
    end

    vals = circshift(vals, [-1 0]);
    vals(lastValIndex) = val;

    mean_val = mean(vals(1:lastValIndex,:));
    if lastValIndex < mov_length
        lastValIndex = lastValIndex + 1;
    end
end

== matlab function aquabot_main/Map builder/MATLAB Function1 ==
  data: scan_msg input; map_matrix output; pose_x input; pose_y input; yaw input
function map_matrix= fcn(scan_msg, pose_x, pose_y, yaw)
    ranges = scan_msg.ranges;
    ranges(ranges==inf) = NaN;
    angles = transpose(linspace(scan_msg.angle_min, scan_msg.angle_max, length(ranges)));

    map = binaryOccupancyMap(700, 700,1);
    map.GridOriginInLocal = -[diff(map.XWorldLimits) diff(map.YWorldLimits)]/2;
    insertRay(map, [pose_x pose_y yaw], ranges, angles, 130);
    map_matrix = map.occupancyMatrix();
end
